simulink model "sim21"  (R2022a)
settings: Solver=ode23  StartTime=0.0  StopTime=1  MaxStep=1e-3  MinStep=1e-11  AbsTol=1e-7  EnableMultiTasking=on
values from neighbouring files (symbols this model uses):
  PAR = [0.302 13.08 0.302 0.087 0.228 1.662 4]    [parametros_maquina.m]
  REF = [w wb]    [parametros_maquina.m]
  v_max = sqrt(2)*V1    [parametros_maquina.m]
  w = 2*pi*60    (= 376.991118431)    [parametros_maquina.m]
  XINIT = [0 0 0 0 0]    [parametros_maquina.m]
libraries: powerlib_extras x1
settings Model: Creator=Alberto  LastModifiedBy=Usuario
settings SolverCC: AutoScaleAbsTol=off  AlgebraicLoopSolver=TrustRegion
settings DataIOCC: LimitDataPoints=on  SaveFormat=Array  SignalLoggingSaveFormat=ModelDataLogs  ReturnWorkspaceOutputs=off  SignalLoggingName=sigsOut
settings OptimizationCC: ExpressionDepthLimit=2147483647  LifeSpan=inf
settings DebuggingCC: SaveWithParameterizedLinksMsg=none  UnderspecifiedInitializationDetection=Classic  MergeDetectMultiDrivingBlocksExec=none  SignalResolutionControl=TryResolveAllWithWarning  MultiTaskDSMMsg=warning  MultiTaskCondExecSysMsg=none  FcnCallInpInsideContextMsg=warning  UnconnectedInputMsg=warning  UnconnectedOutputMsg=warning  UnconnectedLineMsg=warning  StateNameClashWarn=warning  SFUnexpectedBacktrackingDiag=warning  SFNoUnconditionalDefaultTransitionDiag=warning  SFExecutionAtInitializationDiag=none  SFMachineParentedDataDiag=warning  ArithmeticOperatorsInVariantConditions=warning
settings HardwareCC: ProdBitPerPointer=32  ProdBitPerSizeT=32  ProdBitPerPtrDiffT=32  ProdLargestAtomicFloat=None  ProdIntDivRoundTo=Undefined  ProdEndianess=Unspecified  ProdWordSize=32  ProdHWDeviceType=32-bit Generic  TargetUnknown=on
settings ModelReferenceCC: PropagateSignalLabelsOutOfModel=off
settings SFSimCC: SimUseLocalCustomCode=off  CustomCodeUndefinedFunction=UseInterfaceOnly
settings RTWCC: RTWUseLocalCustomCode=off
settings CodeAppCC: StateflowObjectComments=on
settings GRTTargetCC: TargetLangStandard=C89/C90 (ANSI)  CombineOutputUpdateFcns=off  GRTInterface=on
settings ConfigComp: CovMetricSettings=dw  CovSaveCumulativeToWorkspaceVar=on  CovSaveSingleToWorkspaceVar=on  CovExternalEMLEnable=off

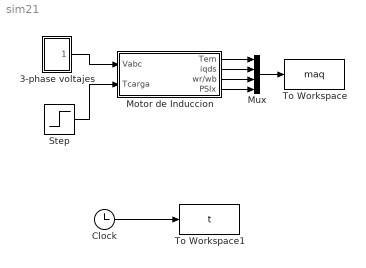
== system sim21 ==
  3-phase voltajes : Subsystem
  Clock : Clock
  Motor de Induccion : Subsystem
  Mux : Mux
  Step : Step  Time=0  After=0  SampleTime=0
  To Workspace : ToWorkspace  VariableName=maq  SampleTime=-1
  To Workspace1 : ToWorkspace  VariableName=t  SampleTime=-1
  wires:
  Mux/1 -> To Workspace/1
  Motor de Induccion/1(Tem) -> Mux/1
  Motor de Induccion/2(iqds) -> Mux/2
  Motor de Induccion/3(wr/wb) -> Mux/3
  Motor de Induccion/4(PSIx) -> Mux/4
  Step/1 -> Motor de Induccion/2(Tcarga)
  3-phase voltajes/1(Vabc) -> Motor de Induccion/1(Vabc)
  Clock/1 -> To Workspace1/1

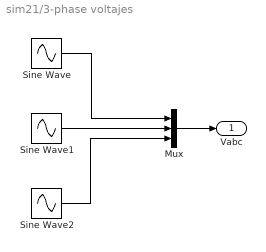
== system sim21/3-phase voltajes ==
  Mux : Mux  Inputs=3
  Sine Wave : Sin  Amplitude=v_max  Frequency=2*pi*60  SampleTime=0
  Sine Wave1 : Sin  Amplitude=v_max  Frequency=2*pi*60  Phase=-2*pi/3  SampleTime=0
  Sine Wave2 : Sin  Amplitude=v_max  Frequency=2*pi*60  Phase=2*pi/3  SampleTime=0
  Vabc : Outport
  wires:
  Sine Wave/1 -> Mux/1
  Sine Wave1/1 -> Mux/2
  Sine Wave2/1 -> Mux/3
  Mux/1 -> Vabc/1

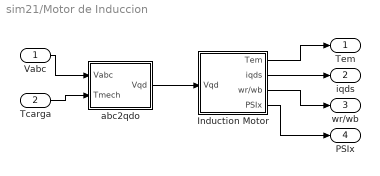
== system sim21/Motor de Induccion ==
  Vabc : Inport
  Tcarga : Inport  Port=2
  Induction Motor : Subsystem
  abc2qdo : Subsystem
      settings: AttributesFormatString=%<IOSignalStrings>
  Tem : Outport
  iqds : Outport  Port=2
  wr/wb : Outport  Port=3
  PSIx : Outport  Port=4
  wires:
  abc2qdo/1(Vqd) -> Induction Motor/1(Vqd)
  Tcarga/1 -> abc2qdo/2(Tmech)
  Vabc/1 -> abc2qdo/1(Vabc)
  Induction Motor/1(Tem) -> Tem/1
  Induction Motor/2(iqds) -> iqds/1
  Induction Motor/3(wr/wb) -> wr/wb/1
  Induction Motor/4(PSIx) -> PSIx/1

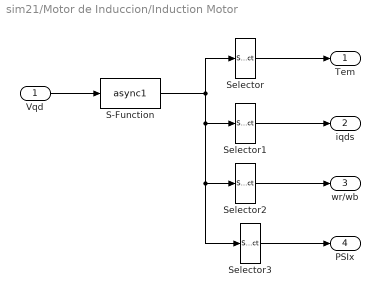
== system sim21/Motor de Induccion/Induction Motor ==
  Vqd : Inport
  S-Function : S-Function  FunctionName=async1  Parameters=XINIT,PAR,REF  SFunctionDeploymentMode=off  EnableBusSupport=off
  Selector : Selector  InputPortWidth=8  IndexOptions=Index vector (dialog)  Indices=[1]  OutputSizes=1
  Selector1 : Selector  InputPortWidth=8  IndexOptions=Index vector (dialog)  Indices=[3 4]  OutputSizes=1
  Selector2 : Selector  InputPortWidth=8  IndexOptions=Index vector (dialog)  Indices=[2]  OutputSizes=1
  Selector3 : Selector  InputPortWidth=8  IndexOptions=Index vector (dialog)  Indices=[5 6 7 8]  OutputSizes=1
  Tem : Outport
  iqds : Outport  Port=2
  wr/wb : Outport  Port=3
  PSIx : Outport  Port=4
  wires:
  S-Function/1 -> Selector/1, Selector1/1, Selector2/1, Selector3/1
  Selector/1 -> Tem/1
  Selector1/1 -> iqds/1
  Selector2/1 -> wr/wb/1
  Selector3/1 -> PSIx/1
  Vqd/1 -> S-Function/1

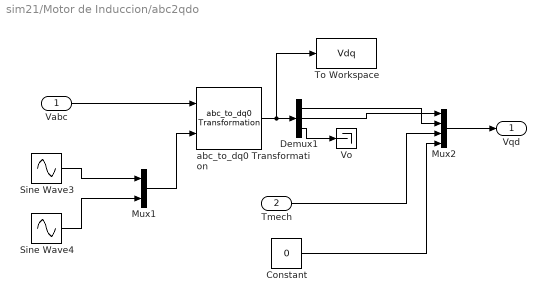
== system sim21/Motor de Induccion/abc2qdo ==
  Vabc : Inport
  Tmech : Inport  Port=2
  Constant : Constant  Value=0
  Demux1 : Demux  Outputs=3
      settings: DisplayOption=none
  Mux1 : Mux  Inputs=2
  Mux2 : Mux
  Sine Wave3 : Sin  Frequency=w  SampleTime=0
  Sine Wave4 : Sin  Frequency=w  Phase=pi/2  SampleTime=0
  To Workspace : ToWorkspace  VariableName=Vdq  SampleTime=-1
  Vo : Terminator
  abc_to_dq0 Transformation : powerlib_extras/Measurements/abc_to_dq0 Transformation
      settings: SourceProductBaseCode=PS
  Vqd : Outport
  wires:
  Sine Wave3/1 -> Mux1/1
  Sine Wave4/1 -> Mux1/2
  Mux1/1 -> abc_to_dq0 Transformation/2
  abc_to_dq0 Transformation/1 -> Demux1/1, To Workspace/1
  Tmech/1 -> Mux2/3
  Demux1/3 -> Vo/1
  Constant/1 -> Mux2/4
  Vabc/1 -> abc_to_dq0 Transformation/1
  Mux2/1 -> Vqd/1
  Demux1/2 -> Mux2/1
  Demux1/1 -> Mux2/2
